simulink model "teste_simples"  (R2012b)
settings: Solver=ode45  StartTime=0.0  StopTime=6.5  RelTol=1e-3
undefined symbols (not defined in the file or in its folder): sigbuilder_block
libraries: simulink x2
settings Model: Creator=Juliano  LastModifiedBy=Juliano

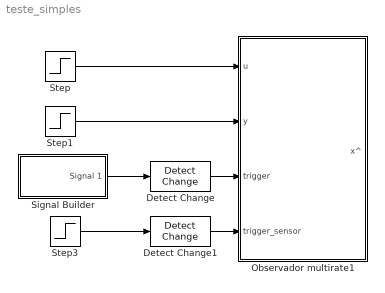
== system teste_simples ==
  Detect Change : simulink/Logic and Bit Operations/Detect Change  vinit=0  InputProcessing=Inherited  OutDataTypeStr=boolean
  Detect Change1 : simulink/Logic and Bit Operations/Detect Change  vinit=0  InputProcessing=Inherited  OutDataTypeStr=boolean
  Observador multirate1 : Subsystem
  Signal Builder : Subsystem  Tag=STV Subsys  LoadFcn=sigbuilder_block('load');  StartFcn=sigbuilder_block('start');  StopFcn=sigbuilder_block('stop');  ClipboardFcn=sigbuilder_block('clipboard');  mask(Sigbuilder block){}
      mask help: Simulink:masks:SigbuilderBlock_MD
      mask init:
      | if ~strcmp(get_param(bdroot(gcbh),'SimulationStatus'),'stopped') tuvar = sigbuilder_block('maskInit'); end
      settings: CopyFcn=sigbuilder_block('copy');  DeleteFcn=sigbuilder_block('delete');  ModelCloseFcn=sigbuilder_block('modelClose');  PreSaveFcn=sigbuilder_block('preSave');  PauseFcn=sigbuilder_block('pause');  ContinueFcn=sigbuilder_block('continue');  NameChangeFcn=sigbuilder_block('namechange');  OpenFcn=sigbuilder_block('open',[437.25 199.5 550.5 399.75 ]);  CloseFcn=sigbuilder_block('close');
      mask Display: plot(0, 0, 100, 100,[2, 2, 32, 32, 2], [68, 8, 8, 68, 68],[32, 2], [38, 38], [32, 19, 2],[53, 60, 44], [32, 17, 17, 2],[16, 16, 31, 31]);txt = getActiveGroup(gcbh);text(2, 100, txt,'verticalAlignment', 'top');
  Step : Step  Time=0  After=10  SampleTime=0
  Step1 : Step  Time=0  After=20  SampleTime=0
  Step3 : Step  Time=2.5  SampleTime=0
  wires:
  Step/1 -> Observador multirate1/1(u)
  Step1/1 -> Observador multirate1/2(y)
  Detect Change/1 -> Observador multirate1/3(trigger)
  Signal Builder/1(Signal 1) -> Detect Change/1
  Detect Change1/1 -> Observador multirate1/4(trigger_sensor)
  Step3/1 -> Detect Change1/1

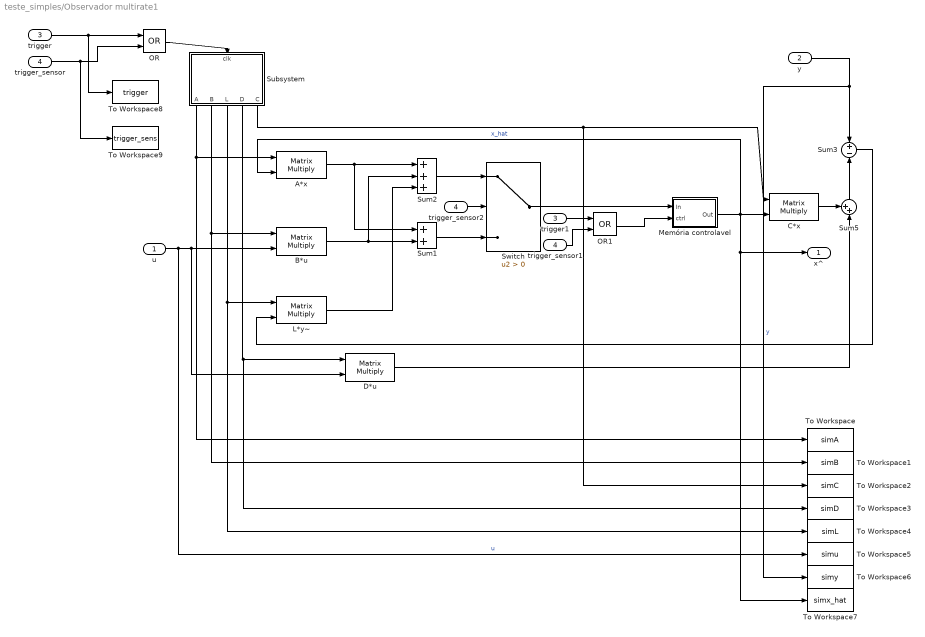
== system teste_simples/Observador multirate1 ==
  u : Inport
  y : Inport  Port=2
  trigger : Inport  Port=3
  trigger_sensor : Inport  Port=4
  A*x : Product  Multiplication=Matrix(*)  RndMeth=Zero
  B*u : Product  Multiplication=Matrix(*)  RndMeth=Zero
  C*x : Product  Multiplication=Matrix(*)  RndMeth=Zero
  D*u : Product  Multiplication=Matrix(*)  RndMeth=Zero
  L*y~ : Product  Multiplication=Matrix(*)  RndMeth=Zero
  Memória controlavel : Subsystem
  OR : Logic  Operator=OR  AllPortsSameDT=off  OutDataTypeStr=boolean
  OR1 : Logic  Operator=OR  AllPortsSameDT=off  OutDataTypeStr=boolean
  Subsystem : Subsystem
  Sum1 : Sum
  Sum2 : Sum  Inputs=+++
  Sum3 : Sum  Inputs=+-
  Sum5 : Sum  Inputs=++|
  Switch : Switch  Criteria=u2 > Threshold
  To Workspace : ToWorkspace  VariableName=simA  SampleTime=-1
  To Workspace1 : ToWorkspace  VariableName=simB  SampleTime=-1
  To Workspace2 : ToWorkspace  VariableName=simC  SampleTime=-1
  To Workspace3 : ToWorkspace  VariableName=simD  SampleTime=-1
  To Workspace4 : ToWorkspace  VariableName=simL  SampleTime=-1
  To Workspace5 : ToWorkspace  VariableName=simu  SampleTime=-1
  To Workspace6 : ToWorkspace  VariableName=simy  SampleTime=-1
  To Workspace7 : ToWorkspace  VariableName=simx_hat  SampleTime=-1
  To Workspace8 : ToWorkspace  VariableName=trigger  SampleTime=-1
  To Workspace9 : ToWorkspace  VariableName=trigger_sens  SampleTime=-1
  trigger1 : InportShadow  Port=3
  trigger_sensor1 : InportShadow  Port=4
  trigger_sensor2 : InportShadow  Port=4
  x^ : Outport
  wires:
  Memória controlavel/1(Out) -> A*x/2, C*x/2, To Workspace7/1, x^/1  "x_hat"
  C*x/1 -> Sum5/1
  u/1 -> To Workspace5/1, B*u/2, D*u/2  "u"
  D*u/1 -> Sum5/2
  Subsystem/1(A) -> To Workspace/1, A*x/1
  Subsystem/2(B) -> To Workspace1/1, B*u/1
  Subsystem/3(L) -> To Workspace4/1, L*y~/1
  Subsystem/4(D) -> To Workspace3/1, D*u/1
  A*x/1 -> Sum2/1, Sum1/1
  B*u/1 -> Sum2/2, Sum1/2
  Sum2/1 -> Switch/1
  Sum1/1 -> Switch/3
  Switch/1 -> Memória controlavel/1(In)
  Subsystem/5(C) -> To Workspace2/1, C*x/1
  y/1 -> To Workspace6/1, Sum3/1  "y"
  Sum5/1 -> Sum3/2
  Sum3/1 -> L*y~/2
  trigger1/1 -> OR1/1
  trigger_sensor1/1 -> OR1/2
  OR1/1 -> Memória controlavel/2(ctrl)
  trigger/1 -> To Workspace8/1, OR/1
  trigger_sensor/1 -> To Workspace9/1, OR/2
  OR/1 -> Subsystem/1(clk)
  trigger_sensor2/1 -> Switch/2
  L*y~/1 -> Sum2/3

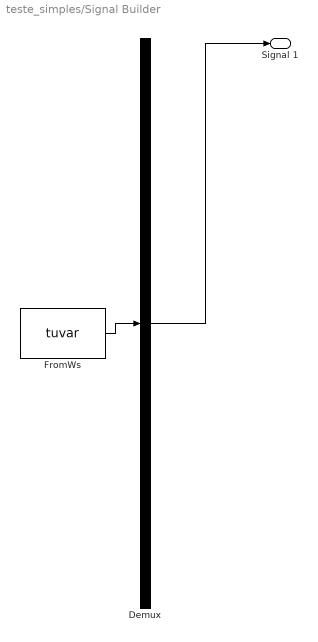
== system teste_simples/Signal Builder ==
  Demux : Demux  Tag=STV Demux  Outputs=1
  FromWs : FromWorkspace  Tag=STV FromWs  VariableName=tuvar  SampleTime=0
      SigBuilderData=|
      | common.afterFinalStr = 'Extrapolate'
      | common.sampleTime = 0
      | dataSet.timeRange = [0 10]
      | dataSet.name = 'Group 1'
      | sbobj.Groups.Name = 'Group 1'
      | sbobj.Groups.Signals.Name = 'Signal 1'
      | sbobj.Groups.Signals.XData = [0 1 1 2 2 5.5 5.5 10]
      | sbobj.Groups.Signals.YData = [0 0 1 1 0 0 1 1]
  Signal 1 : Outport  Tag=STV Outport
  wires:
  Demux/1 -> Signal 1/1
  FromWs/1 -> Demux/1

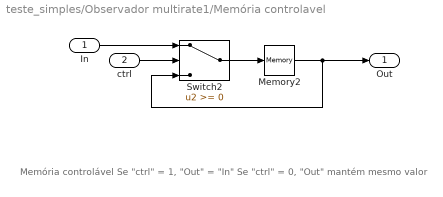
== system teste_simples/Observador multirate1/Memória controlavel ==
  note: Memória controlável
      |
      | Se "ctrl" = 1, "Out" = "In"
      | Se "ctrl" = 0, "Out" mantém mesmo valor
  In : Inport
  ctrl : Inport  Port=2
  Memory2 : Memory
  Switch2 : Switch
  Out : Outport
  wires:
  Switch2/1 -> Memory2/1
  Memory2/1 -> Out/1, Switch2/3
  ctrl/1 -> Switch2/2
  In/1 -> Switch2/1

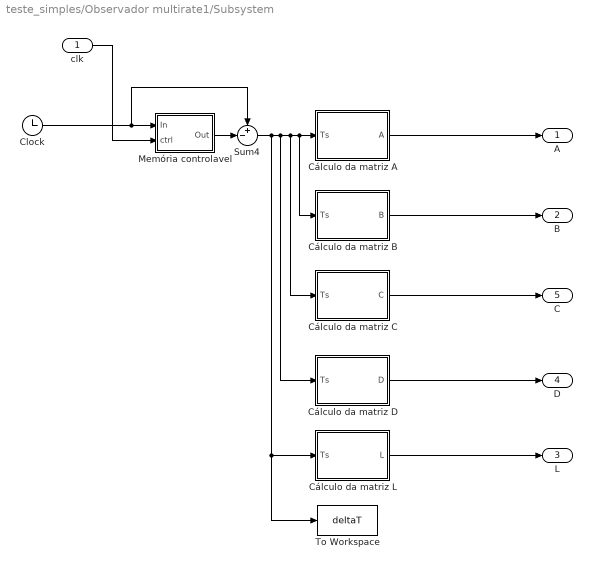
== system teste_simples/Observador multirate1/Subsystem ==
  clk : Inport
  Clock : Clock
  Cálculo da matriz A : MATLAB Function  TreatAsAtomicUnit=on
  Cálculo da matriz B : MATLAB Function  TreatAsAtomicUnit=on
  Cálculo da matriz C : MATLAB Function  TreatAsAtomicUnit=on
  Cálculo da matriz D : MATLAB Function  TreatAsAtomicUnit=on
  Cálculo da matriz L : MATLAB Function  TreatAsAtomicUnit=on
  Memória controlavel : Subsystem
  Sum4 : Sum  Inputs=+-|
  To Workspace : ToWorkspace  VariableName=deltaT  SampleTime=-1
  A : Outport
  B : Outport  Port=2
  L : Outport  Port=3
  D : Outport  Port=4
  C : Outport  Port=5
  wires:
  Clock/1 -> Sum4/1, Memória controlavel/1(In)
  Memória controlavel/1(Out) -> Sum4/2
  clk/1 -> Memória controlavel/2(ctrl)
  Sum4/1 -> To Workspace/1, Cálculo da matriz L/1(Ts), Cálculo da matriz D/1(Ts), Cálculo da matriz C/1(Ts), Cálculo da matriz B/1(Ts), Cálculo da matriz A/1(Ts)
  Cálculo da matriz L/1(L) -> L/1
  Cálculo da matriz D/1(D) -> D/1
  Cálculo da matriz C/1(C) -> C/1
  Cálculo da matriz B/1(B) -> B/1
  Cálculo da matriz A/1(A) -> A/1

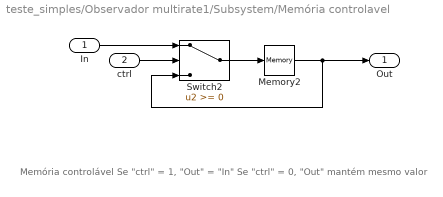
== system teste_simples/Observador multirate1/Subsystem/Memória controlavel ==
  note: Memória controlável
      |
      | Se "ctrl" = 1, "Out" = "In"
      | Se "ctrl" = 0, "Out" mantém mesmo valor
  In : Inport
  ctrl : Inport  Port=2
  Memory2 : Memory
  Switch2 : Switch
  Out : Outport
  wires:
  In/1 -> Switch2/1
  ctrl/1 -> Switch2/2
  Memory2/1 -> Switch2/3, Out/1
  Switch2/1 -> Memory2/1

== matlab function teste_simples/Observador multirate1/Subsystem/Cálculo da matriz A ==
  data: Ts input; A output
function A = fcn(Ts)
%#codegen

A = [1-0.2*Ts 0 ; Ts 1];

== matlab function teste_simples/Observador multirate1/Subsystem/Cálculo da matriz B ==
  data: Ts input; B output
function B = fcn(Ts)
%#codegen

B = [10*Ts ; 0];

== matlab function teste_simples/Observador multirate1/Subsystem/Cálculo da matriz C ==
  data: Ts input; C output
function C = fcn(Ts)
%#codegen

C = [0 1];

== matlab function teste_simples/Observador multirate1/Subsystem/Cálculo da matriz D ==
  data: Ts input; D output
function D = fcn(Ts)
%#codegen

D = [0];

== matlab function teste_simples/Observador multirate1/Subsystem/Cálculo da matriz L ==
  data: Ts input; L output
function L = fcn(Ts)
%#codegen

L = [-0.18+0.2/Ts+0.04*Ts ; 0.9-0.2*Ts];
